simulink model "two"  (R2018a)
settings: Solver=VariableStepAuto  StartTime=0.0  StopTime=10.0  RelTol=1e-3
settings Model: Creator=asish  LastModifiedBy=asish

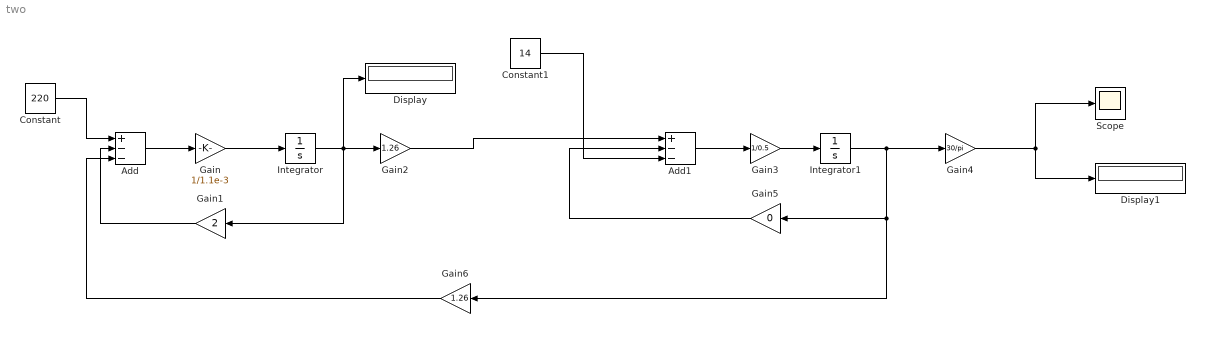
== system two ==
  Add : Sum  Inputs=+--
  Add1 : Sum  Inputs=+--
  Constant : Constant  Value=220
  Constant1 : Constant  Value=14
  Display : Display
  Display1 : Display
  Gain : Gain  Gain=1/1.1e-3
  Gain1 : Gain  Gain=2
  Gain2 : Gain  Gain=1.26
  Gain3 : Gain  Gain=1/0.5
  Gain4 : Gain  Gain=30/pi
  Gain5 : Gain  Gain=0
  Gain6 : Gain  Gain=1.26
  Integrator : Integrator
  Integrator1 : Integrator
  Scope : Scope
  wires:
  Gain/1 -> Integrator/1
  Constant/1 -> Add/1
  Add/1 -> Gain/1
  Integrator/1 -> Display/1, Gain2/1, Gain1/1
  Gain1/1 -> Add/2
  Gain2/1 -> Add1/1
  Constant1/1 -> Add1/3
  Add1/1 -> Gain3/1
  Gain3/1 -> Integrator1/1
  Integrator1/1 -> Gain6/1, Gain5/1, Gain4/1
  Gain4/1 -> Display1/1, Scope/1
  Gain5/1 -> Add1/2
  Gain6/1 -> Add/3
